simulink model "Part_b"  (R2021b)
settings: Solver=ode45  StartTime=0  StopTime=100  RelTol=1e-3
settings Model: Creator=jimd  LastModifiedBy=jimd

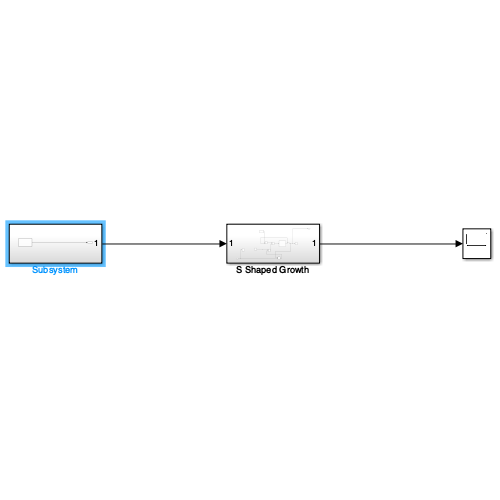
[thumbnail: Simulink's stored preview of the top-level diagram]
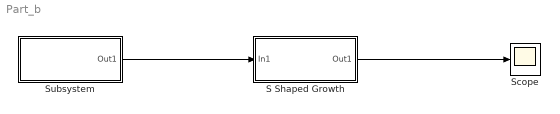
== system Part_b ==
  S Shaped Growth : Subsystem
  Scope : Scope
  Subsystem : Subsystem
  wires:
  Subsystem/1(Out1) -> S Shaped Growth/1(In1)
  S Shaped Growth/1(Out1) -> Scope/1

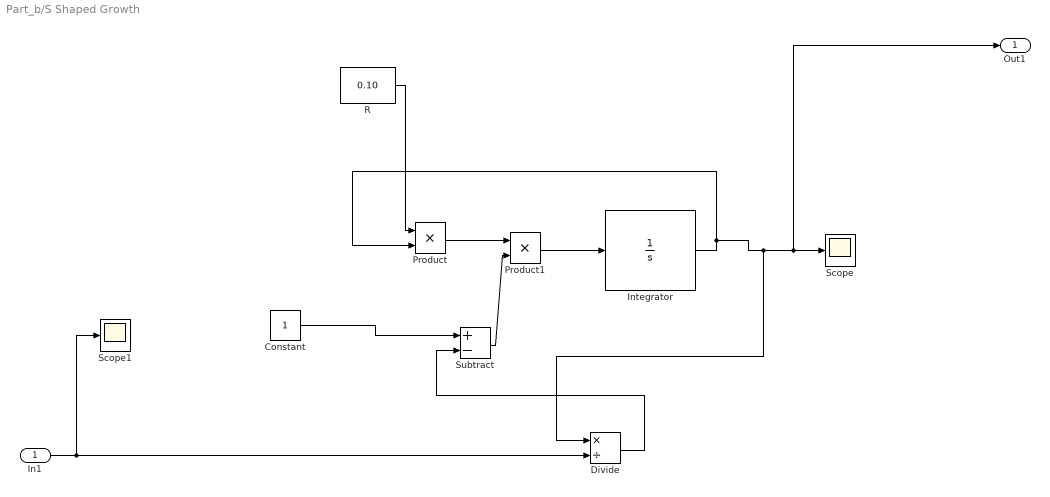
== system Part_b/S Shaped Growth ==
  In1 : Inport
  Constant : Constant
  Divide : Product  Inputs=*/
  Integrator : Integrator  InitialCondition=1000
  Product : Product
  Product1 : Product
  R : Constant  Value=0.10
  Scope : Scope
  Scope1 : Scope
  Subtract : Sum  Inputs=+-
  Out1 : Outport
  wires:
  Product/1 -> Product1/1
  R/1 -> Product/1
  Integrator/1 -> Product/2, Divide/1, Out1/1, Scope/1
  Product1/1 -> Integrator/1
  Subtract/1 -> Product1/2
  Constant/1 -> Subtract/1
  Divide/1 -> Subtract/2
  In1/1 -> Divide/2, Scope1/1

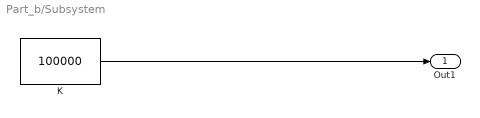
== system Part_b/Subsystem ==
  K : Constant  Value=100000
  Out1 : Outport
  wires:
  K/1 -> Out1/1
